simulink model "Motor_Controller"  (R2023b)
settings: Solver=VariableStepAuto  StartTime=0.0  StopTime=10.0  RelTol=1e-3
settings Model: Creator=siva kumar  LastModifiedBy=siva kumar

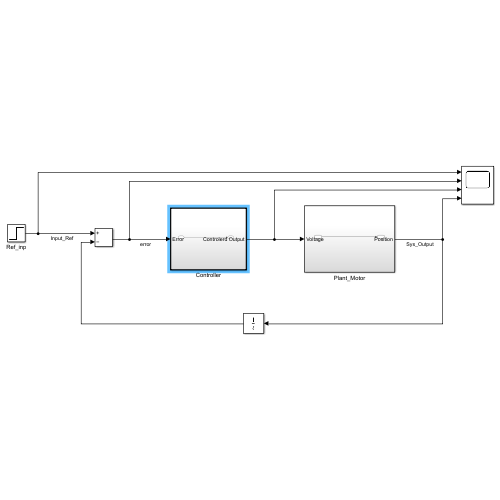
[thumbnail: Simulink's stored preview of the top-level diagram]
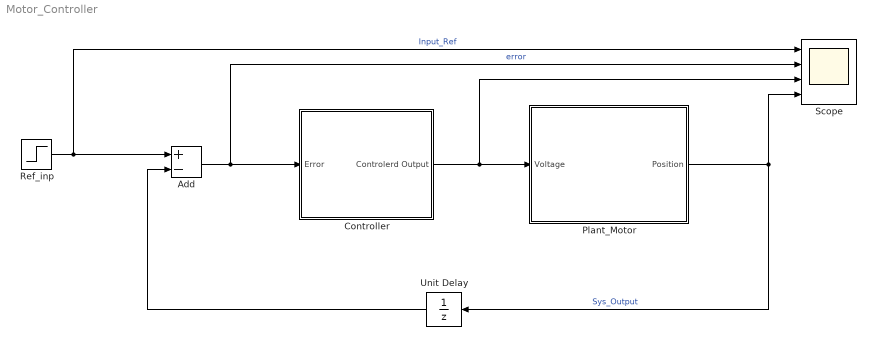
== system Motor_Controller ==
  Add : Sum  Inputs=+-
  Controller : Subsystem  TreatAsAtomicUnit=on
  Plant_Motor : Subsystem
  Ref_inp : Step  SampleTime=0
  Scope : Scope  NumInputPorts=4
  Unit Delay : UnitDelay  SampleTime=-1  HasFrameUpgradeWarning=on
  wires:
  Controller/1(Controlerd Output) -> Scope/3, Plant_Motor/1(Voltage)
  Add/1 -> Scope/2, Controller/1(Error)  "error"
  Plant_Motor/1(Position) -> Scope/4, Unit Delay/1  "Sys_Output"
  Ref_inp/1 -> Scope/1, Add/1  "Input_Ref"
  Unit Delay/1 -> Add/2

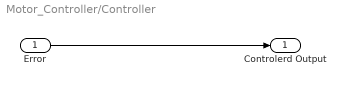
== system Motor_Controller/Controller ==
  Error : Inport
  Controlerd Output : Outport
  wires:
  Error/1 -> Controlerd Output/1

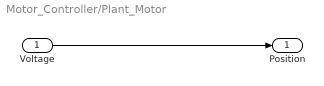
== system Motor_Controller/Plant_Motor ==
  Voltage : Inport
  Position : Outport
  wires:
  Voltage/1 -> Position/1
